simulink model "A1"  (R2024a)
settings: Solver=ode4  StartTime=0.0  StopTime=60  FixedStep=0.4  RelTol=1e-3
values from neighbouring files (symbols this model uses):
  A = [0,1;-1/4,0]    [A1_mat.m]
  b = [0;1/4]    [A1_mat.m]
  c = [1,0]    [A1_mat.m]
  d = 0    [A1_mat.m]
settings Model: Creator=Flipper  LastModifiedBy=Flipper

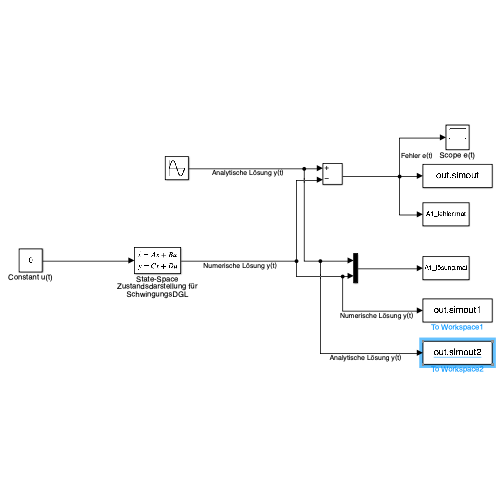
[thumbnail: Simulink's stored preview of the top-level diagram]
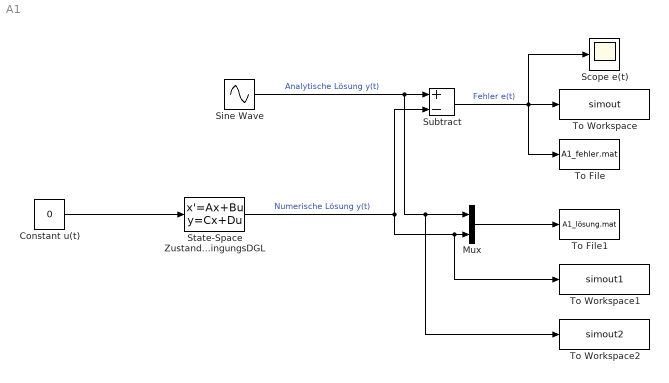
== system A1 ==
  Constant u(t) : Constant  Value=0
  Mux : Mux  Inputs=2
  Scope e(t) : Scope
  Sine Wave : Sin  Amplitude=2  Frequency=1/2  SampleTime=0
  State-Space Zustandsdarstellung für SchwingungsDGL : StateSpace  A=A  B=b  C=c  D=d  InitialCondition=[0;1]
  Subtract : Sum  Inputs=+-
  To File : ToFile  Filename=A1_fehler.mat  SaveFormat=Timeseries
  To File1 : ToFile  Filename=A1_lösung.mat  SaveFormat=Timeseries
  To Workspace : ToWorkspace  VariableName=simout  SaveFormat=Timeseries  SampleTime=-1
  To Workspace1 : ToWorkspace  VariableName=simout1  SaveFormat=Timeseries  SampleTime=-1
  To Workspace2 : ToWorkspace  VariableName=simout2  SaveFormat=Timeseries  SampleTime=-1
  wires:
  Mux/1 -> To File1/1
  Constant u(t)/1 -> State-Space Zustandsdarstellung für SchwingungsDGL/1
  Subtract/1 -> To Workspace/1, Scope e(t)/1, To File/1  "Fehler e(t)"
  State-Space Zustandsdarstellung für SchwingungsDGL/1 -> To Workspace1/1, Mux/2, Subtract/2  "Numerische Lösung y(t)"
  Sine Wave/1 -> To Workspace2/1, Mux/1, Subtract/1  "Analytische Lösung y(t)"
